simulink model "carSimC_xyth"  (R2020b)
settings: Solver=FixedStepAuto  StartTime=0.0  StopTime=20  FixedStep=1e-2  MaxStep=1e-2  RelTol=1e-3  EnableMultiTasking=on
libraries: simulink x3
settings Model: Creator=hp  LastModifiedBy=11634
settings SolverCC: AlgebraicLoopSolver=LineSearch
settings DataIOCC: LimitDataPoints=on  SaveFormat=Array  SignalLoggingSaveFormat=ModelDataLogs  ReturnWorkspaceOutputs=off  SignalLoggingName=sigsOut
settings OptimizationCC: ExpressionDepthLimit=2147483647  InitFltsAndDblsToZero=on  LifeSpan=inf
settings DebuggingCC: SaveWithParameterizedLinksMsg=none  UnderspecifiedInitializationDetection=Classic  MergeDetectMultiDrivingBlocksExec=none  SignalResolutionControl=TryResolveAllWithWarning  MultiTaskDSMMsg=warning  MultiTaskCondExecSysMsg=none  FcnCallInpInsideContextMsg=warning  StateNameClashWarn=warning  SFUnexpectedBacktrackingDiag=warning  SFNoUnconditionalDefaultTransitionDiag=warning  SFExecutionAtInitializationDiag=none  ArithmeticOperatorsInVariantConditions=warning
settings HardwareCC: ProdBitPerPointer=32  ProdBitPerSizeT=32  ProdBitPerPtrDiffT=32  ProdLargestAtomicFloat=None  ProdIntDivRoundTo=Undefined  ProdEndianess=Unspecified  ProdWordSize=32  ProdHWDeviceType=32-bit Generic  TargetUnknown=on
settings ModelReferenceCC: PropagateSignalLabelsOutOfModel=off
settings SFSimCC: SimUseLocalCustomCode=off  CustomCodeUndefinedFunction=UseInterfaceOnly
settings RTWCC: RTWUseLocalCustomCode=off
settings CodeAppCC: StateflowObjectComments=on
settings GRTTargetCC: TargetFcnLib=ansi_tfl_tmw.mat  TargetLangStandard=C89/C90 (ANSI)  CombineOutputUpdateFcns=off  GRTInterface=on
settings ConfigComp: CovMetricSettings=dw  CovSaveCumulativeToWorkspaceVar=on  CovSaveSingleToWorkspaceVar=on  CovExternalEMLEnable=off

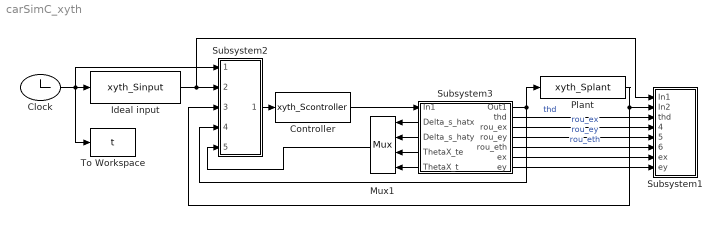
== system carSimC_xyth ==
  Clock : Clock
  Controller : S-Function  FunctionName=xyth_Scontroller  SFunctionDeploymentMode=off  EnableBusSupport=off
  Ideal input : S-Function  FunctionName=xyth_Sinput  SFunctionDeploymentMode=off  EnableBusSupport=off
  Mux1 : Mux
  Plant : S-Function  FunctionName=xyth_Splant  SFunctionDeploymentMode=off  EnableBusSupport=off
  Subsystem1 : Subsystem
  Subsystem2 : Subsystem
  Subsystem3 : Subsystem
      settings: PortSchema="{\"entries\":[{\"content\":{\"sides\":[{\"content\":{\"connectorIds\":[\"In1\",\"Out8\",\"Out9\",\"Out10\",\"Out11\"]},\"type\":\"ConnectorPlacement.EquallySpacedRectSide\",\"uuid\":\"744a0110-5fd8-42fe-8157-adca7d82f44f\"},{\"content\":{\"connectorIds\":[\"Out1\",\"Out2\",\"Out3\",\"Out4\",\"Out5\",\"Out6\",\"Out7\"],\"side\":\"RIGHT\"},\"type\":\"ConnectorPlacement.EquallySpacedRectSide\",\"uuid\":\"3f0d3f71-8b45-482e-9cbd-bb0c457f5e09\"},{\"content\":{\"connectorIds\":[],\"side\":\"TOP\"},\"type\":\"ConnectorPlacement.EquallySpacedRectSide\",\"uuid\":\"2cc30f63-657e-4255-938f-24588c68dc3e\"},{\"content\":{\"connectorIds\":[],\"side\":\"BOTTOM\"},\"type\":\"ConnectorPlacement.EquallySpacedRectSide\",\"uuid\":\"9eda8ca2-e87f-4aed-b5aa-d74f341b86df\"},{\"content\":{\"connectorIds\":[],\"side\":\"HIDDEN\"},\"type\":\"ConnectorPlacement.EquallySpacedRectSide\",\"uuid\":\"771eac1c-3326-40e1-b7ab-ddc49b193a5b\"}]},\"type\":\"ConnectorPlacement.EquallySpacedConnector\",\"uuid\":\"7b012369-4162-4ea1-939d-d49a3361749e\"}],\"packageUris\":[\"http://schema.mathworks.com/mf0/Connector/R2020b\"],\"version\":\"1.0\"}"
  To Workspace : ToWorkspace  VariableName=t  SampleTime=-1
  wires:
  Plant/1 -> Subsystem2/3(In3), Subsystem1/2(In2)
  Clock/1 -> To Workspace/1, Subsystem2/1(In1), Ideal input/1
  Ideal input/1 -> Subsystem2/2(In2), Subsystem1/1(In1)
  Controller/1 -> Subsystem3/1(In1)
  Subsystem3/2(thd) -> Subsystem1/3(thd)  "thd"
  Subsystem3/3(rou_ex) -> Subsystem1/4(rou_ex)  "rou_ex"
  Subsystem3/4(rou_ey) -> Subsystem1/5(rou_ey)  "rou_ey"
  Subsystem3/5(rou_eth) -> Subsystem1/6(rou_eth)  "rou_eth"
  Subsystem3/6(ex) -> Subsystem1/7(ex)
  Subsystem3/7(ey) -> Subsystem1/8(ey)
  Subsystem3/1(Out1) -> Subsystem2/4(In4), Plant/1
  Subsystem2/1(Out1) -> Controller/1
  Mux1/1 -> Subsystem2/5(In5)
  Subsystem3/9(Delta_s_haty) -> Mux1/2
  Subsystem3/8(Delta_s_hatx) -> Mux1/1
  Subsystem3/11(ThetaX_t) -> Mux1/4
  Subsystem3/10(ThetaX_te) -> Mux1/3

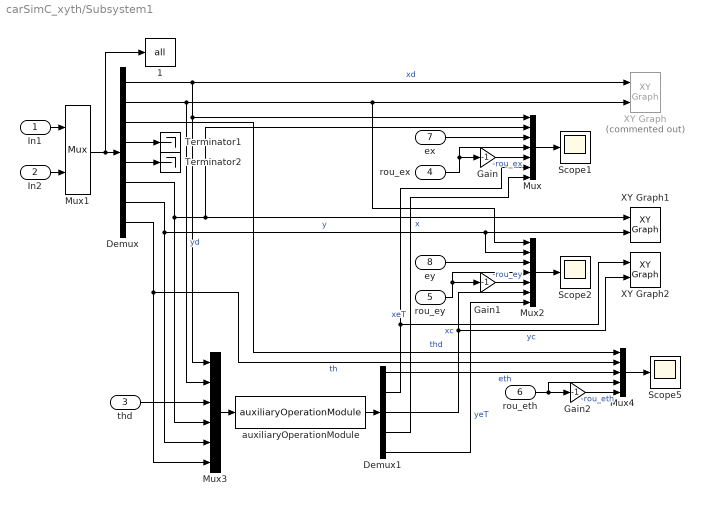
== system carSimC_xyth/Subsystem1 ==
  In1 : Inport
  In2 : Inport  Port=2
  thd : Inport  Port=3
  rou_ex : Inport  Port=4
  rou_ey : Inport  Port=5
  rou_eth : Inport  Port=6
  ex : Inport  Port=7
  ey : Inport  Port=8
  " 1" : ToWorkspace  VariableName=all  SampleTime=-1
  Demux : Demux  Outputs=8
  Demux1 : Demux  Outputs=5
  Gain : Gain  Gain=-1
  Gain1 : Gain  Gain=-1
  Gain2 : Gain  Gain=-1
  Mux : Mux  Inputs=7
  Mux1 : Mux  Inputs=2
  Mux2 : Mux  Inputs=7
  Mux3 : Mux  Inputs=6
  Mux4 : Mux  Inputs=5
  Scope1 : Scope
  Scope2 : Scope
  Scope5 : Scope
  Terminator1 : Terminator
  Terminator2 : Terminator
  XY Graph : simulink/Sinks/XY Graph  Commented=on  xmin=-4  xmax=4  ymin=-4  ymax=4  st=-1
  XY Graph1 : simulink/Sinks/XY Graph  xmin=-4  xmax=4  ymin=-4  ymax=4  st=-1
  XY Graph2 : simulink/Sinks/XY Graph  xmin=-4  xmax=4  ymin=-4  ymax=4  st=-1
  auxiliaryOperationModule : S-Function  FunctionName=auxiliaryOperationModule  SFunctionDeploymentMode=off  EnableBusSupport=off
  wires:
  Demux/1 -> Mux3/1, Mux/1, XY Graph/1  "xd"
  Demux/7 -> Mux3/5, Mux2/2, XY Graph1/2  "y"
  Mux1/1 -> " 1"/1, Demux/1
  rou_eth/1 -> Mux4/4, Gain2/1
  Gain2/1 -> Mux4/5  "-rou_eth"
  Demux/6 -> Mux3/4, XY Graph1/1, Mux/2  "x"
  Mux/1 -> Scope1/1
  Demux/2 -> Mux3/2, XY Graph/2, Mux2/1  "yd"
  Demux/8 -> Mux3/6, Mux4/2  "th"
  Demux1/1 -> Mux4/3  "eth"
  In2/1 -> Mux1/2
  Gain/1 -> Mux/5  "-rou_ex"
  Gain1/1 -> Mux2/5  "-rou_ey"
  Mux2/1 -> Scope2/1
  Mux4/1 -> Scope5/1
  rou_ex/1 -> Gain/1, Mux/4
  Demux/3 -> Mux4/1  "thd"
  In1/1 -> Mux1/1
  thd/1 -> Mux3/3
  rou_ey/1 -> Mux2/4, Gain1/1
  ey/1 -> Mux2/3
  ex/1 -> Mux/3
  auxiliaryOperationModule/1 -> Demux1/1
  Mux3/1 -> auxiliaryOperationModule/1
  Demux1/2 -> Mux/6, XY Graph2/1  "xc"
  Demux1/4 -> Mux/7  "xeT"
  Demux1/3 -> Mux2/6, XY Graph2/2  "yc"
  Demux1/5 -> Mux2/7  "yeT"
  Demux/4 -> Terminator1/1
  Demux/5 -> Terminator2/1

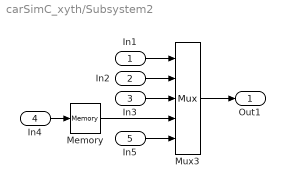
== system carSimC_xyth/Subsystem2 ==
  In1 : Inport
  In2 : Inport  Port=2
  In3 : Inport  Port=3
  In4 : Inport  Port=4
  In5 : Inport  Port=5
  Memory : Memory
  Mux3 : Mux  Inputs=5
  Out1 : Outport
  wires:
  In1/1 -> Mux3/1
  Mux3/1 -> Out1/1
  In2/1 -> Mux3/2
  In3/1 -> Mux3/3
  Memory/1 -> Mux3/4
  In4/1 -> Memory/1
  In5/1 -> Mux3/5

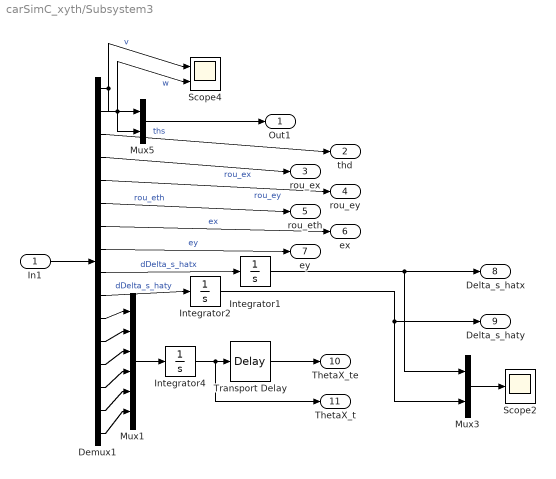
== system carSimC_xyth/Subsystem3 ==
  In1 : Inport
  Demux1 : Demux  Outputs=16
  Integrator1 : Integrator
  Integrator2 : Integrator
  Integrator4 : Integrator
  Mux1 : Mux  Inputs=6
  Mux3 : Mux  Inputs=2
  Mux5 : Mux  Inputs=2
  Scope2 : Scope
  Scope4 : Scope  NumInputPorts=2
  Transport Delay : TransportDelay  DelayTime=0.5  BufferSize=10240
  Out1 : Outport
  thd : Outport  Port=2
  rou_ex : Outport  Port=3
  rou_ey : Outport  Port=4
  rou_eth : Outport  Port=5
  ex : Outport  Port=6
  ey : Outport  Port=7
  Delta_s_hatx : Outport  Port=8
  Delta_s_haty : Outport  Port=9
  ThetaX_te : Outport  Port=10
  ThetaX_t : Outport  Port=11
  wires:
  In1/1 -> Demux1/1
  Demux1/2 -> Scope4/2, Mux5/2  "w"
  Mux5/1 -> Out1/1
  Demux1/1 -> Scope4/1, Mux5/1  "v"
  Demux1/3 -> thd/1  "ths"
  Demux1/4 -> rou_ex/1  "rou_ex"
  Demux1/5 -> rou_ey/1  "rou_ey"
  Demux1/6 -> rou_eth/1  "rou_eth"
  Demux1/8 -> ey/1  "ey"
  Demux1/7 -> ex/1  "ex"
  Demux1/9 -> Integrator1/1  "dDelta_s_hatx"
  Demux1/10 -> Integrator2/1  "dDelta_s_haty"
  Demux1/11 -> Mux1/1
  Demux1/12 -> Mux1/2
  Demux1/13 -> Mux1/3
  Demux1/14 -> Mux1/4
  Demux1/15 -> Mux1/5
  Demux1/16 -> Mux1/6
  Mux1/1 -> Integrator4/1
  Integrator4/1 -> ThetaX_t/1, Transport Delay/1
  Transport Delay/1 -> ThetaX_te/1
  Integrator1/1 -> Mux3/1, Delta_s_hatx/1
  Integrator2/1 -> Mux3/2, Delta_s_haty/1
  Mux3/1 -> Scope2/1
